simulink library "oseklib"  (Simulink 6.0)
settings: Solver=ode45  SolverMode=SingleTasking  StartTime=0.0  StopTime=10.0  RelTol=1e-3
settings Model: Creator=jcarrick  LastModifiedBy=jcarrick  ProdHWDeviceType=Specified
settings DataIOCC: SignalLoggingName=logsOut
settings OptimizationCC: BooleanDataType=off
settings DebuggingCC: CheckExecutionContextPreStartOutputMsg=on  CheckExecutionContextRuntimeOutputMsg=on  SolverPrmCheckMsg=none
settings HardwareCC: ProdHWDeviceType=Specified
settings SFSimCC: SFSimApplyToAllLibs=on  SFSimBuildMode=Incremental

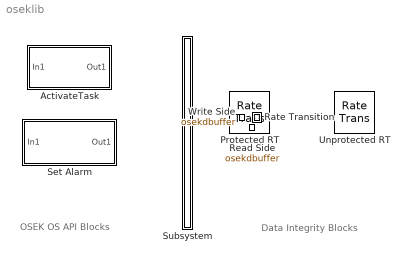
== system oseklib ==
  note: Data Integrity Blocks
  note: OSEK OS API Blocks
  ActivateTask : Subsystem  PropExecContextAcrossSSBoundary=on  mask(OSEK Task Block){taskName=myTask, taskPriority=20, taskStackSize=1024, taskSchedule=FULL}
      mask prompts: taskName "Task name (valid C identifier):"; taskPriority "Task priority (0-255):"; taskStackSize "Stack size (bytes):"; taskSchedule "Preemptive scheduling:"
      mask help: Defines the downstream function-call subsystem as an BCC1 OSEK task. The priority must be unique to the other tasks defined be the model.
      mask init:
      | if ~iscvar(taskName) & (length(taskName) > 0)
      |    errordlg('invalid Task Name, first character must be a letter or underscore and remaining characters must be letters,underscores or numbers.','Task Block Error','replace');
      |    taskName = '';
      | end
      mask Help: helpview([docroot '/toolbox/osek/osek.map'], 'osek_ActivateTask_blkref');
      mask StyleString: edit,edit,edit,popup(FULL|NON)
      mask Display:
      | disp(['       OSEK Task\n','       ''',taskName,''''])
      | port_label('input',1,'Call')
  Protected RT : RateTransition  Deterministic=off
  Rate Transition : Subsystem  PropExecContextAcrossSSBoundary=on  mask(Rate Transition){sample_time=-1}
      mask prompts: sample_time "Sample time:"
      mask help: Converts rate of input signal to specified sample time.
      mask Help: helpview([docroot '/toolbox/osek/osek.map'], 'osek_AsyncRTUnprotected_blkref');
      mask Display: disp(['Unprotected\nOSEK Async\nRate Transition'])
  Read Side : S-Function  FunctionName=osekdbuffer  Parameters=DB_Type, sample_time  mask(Asynchronous Rate Transition: Reader){sample_time=-1}
      mask prompts: sample_time "Sample time:"
      mask help: Double buffer data between asynchronous subsystems/blocks in a model.
      mask init:
      | DB_Type = 'READ';
      mask Help: helpview([docroot '/toolbox/osek/osek.map'], 'osek_AsyncRTReader_blkref');
      mask Display: disp(['OSEK Async\nRate Transition\n(Reader)'])
  Set Alarm : Subsystem  PropExecContextAcrossSSBoundary=on  mask(OSEK Set Alarm Block){alarmName=myAlarm, alarmIncr=100, alarmType=Relative, alarmPlacement=off, alarmCyclic=0}
      mask prompts: alarmName "Alarm name:"; alarmIncr "Increment:"; alarmType "Type:"; alarmPlacement "Call only at startup"; alarmCyclic "Cyclic:"
      mask help: Sets an OSEK Alarm as specified. If 'Startup' placement is selected, the Alarm is set only at model startup.
      mask init:
      | if ~iscvar(alarmName) & (length(alarmName) > 0)
      |    errordlg('invalid Alarm Name, first character must be a letter or underscore and remaining characters must be letters,underscores or numbers.','Task Block Error','replace');
      |    alarmName = '';
      | end
      mask Help: helpview([docroot '/toolbox/osek/osek.map'], 'osek_SetAlarm_blkref');
      mask StyleString: edit,edit,popup(Relative|Absolute),checkbox,edit
      mask CallbackString:
      | |||if strcmp(get_param(gcb,'alarmPlacement'),'on')
      | 	set_param(gcb,'MaskEnables', {'on', 'on', 'on', 'on', 'on'});
      | else
      | 	set_param(gcb,'MaskEnables', {'on', 'on', 'on', 'on', 'off'});
      | end
      | |
      mask Display:
      | disp(['         OSEK Alarm\n','       ''',alarmName,''''])
      | port_label('input',1,'Call')
  Subsystem : Subsystem  PropExecContextAcrossSSBoundary=on
      mask Display: disp('')
  Unprotected RT : RateTransition  Integrity=off
  Write Side : S-Function  FunctionName=osekdbuffer  Parameters=DB_Type, sample_time  mask(Asynchronous Rate Transition: Writer){sample_time=-1}
      mask prompts: sample_time "Sample time:"
      mask help: Double buffer data between asynchronous subsystems/blocks in a model.
      mask init:
      | DB_Type = 'WRITE';
      mask Help: helpview([docroot '/toolbox/osek/osek.map'], 'osek_AsynRTWriter_blkref');
      mask Display: disp(['OSEK Async\nRate Transition\n(Writer)'])

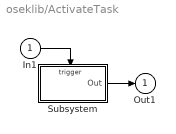
== system oseklib/ActivateTask ==
  In1 : Inport  LatchInput=off
  Subsystem : Subsystem  TreatAsAtomicUnit=on  PropExecContextAcrossSSBoundary=on
      settings: RTWSystemCode=Inline
  Out1 : Outport
  wires:
  In1/1 -> Subsystem/Trigger
  Subsystem/1(Out) -> Out1/1

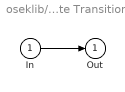
== system oseklib/Rate Transition ==
  In : Inport  Tag=AsyncRateTransition  SampleTime=sample_time  LatchInput=off
  Out : Outport  Tag=AsyncRateTransition  InitialOutput=0
  wires:
  In/1 -> Out/1

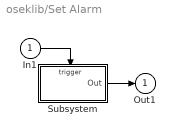
== system oseklib/Set Alarm ==
  In1 : Inport  LatchInput=off
  Subsystem : Subsystem  TreatAsAtomicUnit=on  PropExecContextAcrossSSBoundary=on
      settings: RTWSystemCode=Inline
      mask Type: VxWorks Task Block
  Out1 : Outport
  wires:
  Subsystem/1(Out) -> Out1/1
  In1/1 -> Subsystem/Trigger

== system oseklib/Subsystem ==

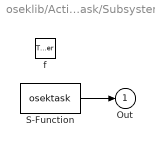
== system oseklib/ActivateTask/Subsystem ==
  f : TriggerPort  TriggerType=function-call
  S-Function : S-Function  FunctionName=osektask  Parameters=taskName, taskPriority, taskStackSize, taskSchedule
  Out : Outport
  wires:
  S-Function/1 -> Out/1

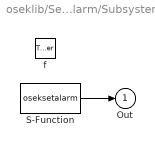
== system oseklib/Set Alarm/Subsystem ==
  f : TriggerPort  TriggerType=function-call
  S-Function : S-Function  FunctionName=oseksetalarm  Parameters=alarmName, alarmIncr, alarmCyclic, alarmType, alarmPlacement
  Out : Outport
  wires:
  S-Function/1 -> Out/1
